simulink model "nonlinearsys"  (Simulink 7.7)
settings: Solver=ode45  StartTime=0.0  StopTime=10.0  RelTol=1e-3
settings Model: Creator=jiannianweng  LastModifiedBy=jiannianweng

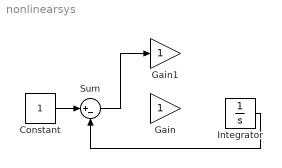
== system nonlinearsys ==
  Constant : Constant
  Gain : Gain
  Gain1 : Gain
  Integrator : Integrator
  Sum : Sum  Inputs=|+-
  wires:
  Constant/1 -> Sum/1
  Integrator/1 -> Sum/2
  Sum/1 -> Gain1/1
